simulink library "dynamic_capacity_server"  (R2019a)
settings: Solver=VariableStepAuto  StartTime=0.0  StopTime=10.0  RelTol=1e-3
undefined symbols (not defined in the file or in its folder): m, n
libraries: $bdroot x9
settings Model: Creator=arsineh  LastModifiedBy=arsineh

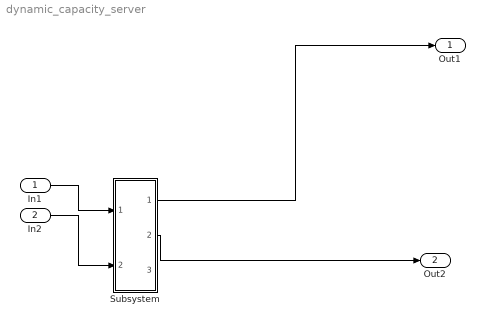
== system dynamic_capacity_server ==
  In1 : Inport
  In2 : Inport  Port=2
  Subsystem : Subsystem
  Out1 : Outport
  Out2 : Outport  Port=2
  wires:
  In1/1 -> Subsystem/1(In1)
  In2/1 -> Subsystem/2(In2)
  Subsystem/1(Out1) -> Out1/1
  Subsystem/2(Out2) -> Out2/1

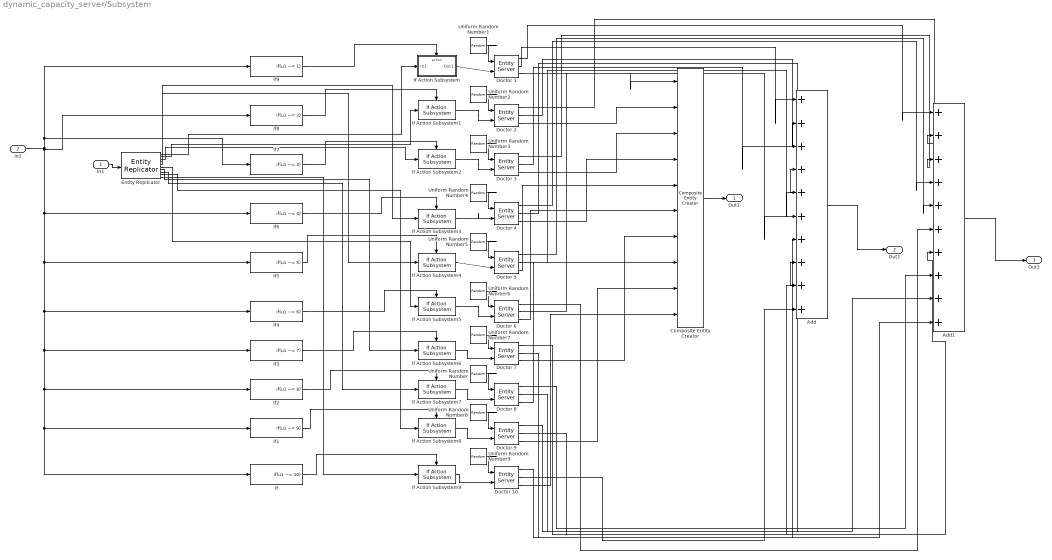
== system dynamic_capacity_server/Subsystem ==
  In1 : Inport
  In2 : Inport  Port=2
  Add : Sum  Inputs=++++++++++
  Add1 : Sum  Inputs=++++++++++
  Composite Entity Creator : CompositeEntityCreator  InputPortMessageModes=m,m,m,m,m,m,m,m,m,m  OutputPortMessageModes=m  NumberInputPorts=10  EntityTypeName=Combined
      settings: InputPortMap=u0,u1,u2,u3,u4,u5,u6,u7,u8,u9
  Doctor 1 : EntityServer  InputPortMessageModes=n,m  OutputPortMessageModes=n,n,m  Capacity=1  ServiceTimeSource=Signal port  ServiceTimeValue=30  ServiceTimeAction=dt = randi([30,60]);  NumberEntitiesDeparted=on  AverageWait=on
      settings: InputPortMap=u0,u2  OutputPortMap=o0,o4,o9
  Doctor 10 : EntityServer  InputPortMessageModes=n,m  OutputPortMessageModes=n,n,m  Capacity=10  ServiceTimeSource=Signal port  ServiceTimeValue=30  ServiceTimeAction=dt = randi([30,60]);  NumberEntitiesDeparted=on  AverageWait=on
      settings: InputPortMap=u0,u2  OutputPortMap=o0,o4,o9
  Doctor 2 : EntityServer  InputPortMessageModes=n,m  OutputPortMessageModes=n,n,m  Capacity=2  ServiceTimeSource=Signal port  ServiceTimeValue=30  ServiceTimeAction=dt = randi([30,60]);  NumberEntitiesDeparted=on  AverageWait=on
      settings: InputPortMap=u0,u2  OutputPortMap=o0,o4,o9
  Doctor 3 : EntityServer  InputPortMessageModes=n,m  OutputPortMessageModes=n,n,m  Capacity=3  ServiceTimeSource=Signal port  ServiceTimeValue=30  ServiceTimeAction=dt = randi([30,60]);  NumberEntitiesDeparted=on  AverageWait=on
      settings: InputPortMap=u0,u2  OutputPortMap=o0,o4,o9
  Doctor 4 : EntityServer  InputPortMessageModes=n,m  OutputPortMessageModes=n,n,m  Capacity=4  ServiceTimeSource=Signal port  ServiceTimeValue=30  ServiceTimeAction=dt = randi([30,60]);  NumberEntitiesDeparted=on  AverageWait=on
      settings: InputPortMap=u0,u2  OutputPortMap=o0,o4,o9
  Doctor 5 : EntityServer  InputPortMessageModes=n,m  OutputPortMessageModes=n,n,m  ServiceTimeSource=Signal port  ServiceTimeValue=30  ServiceTimeAction=dt = randi([30,60]);  NumberEntitiesDeparted=on  AverageWait=on
      settings: InputPortMap=u0,u2  OutputPortMap=o0,o4,o9
  Doctor 6 : EntityServer  InputPortMessageModes=n,m  OutputPortMessageModes=n,n,m  Capacity=6  ServiceTimeSource=Signal port  ServiceTimeValue=30  ServiceTimeAction=dt = randi([30,60]);  NumberEntitiesDeparted=on  AverageWait=on
      settings: InputPortMap=u0,u2  OutputPortMap=o0,o4,o9
  Doctor 7 : EntityServer  InputPortMessageModes=n,m  OutputPortMessageModes=n,n,m  Capacity=7  ServiceTimeSource=Signal port  ServiceTimeValue=30  ServiceTimeAction=dt = randi([30,60]);  NumberEntitiesDeparted=on  AverageWait=on
      settings: InputPortMap=u0,u2  OutputPortMap=o0,o4,o9
  Doctor 8 : EntityServer  InputPortMessageModes=n,m  OutputPortMessageModes=n,n,m  Capacity=8  ServiceTimeSource=Signal port  ServiceTimeValue=30  ServiceTimeAction=dt = randi([30,60]);  NumberEntitiesDeparted=on  AverageWait=on
      settings: InputPortMap=u0,u2  OutputPortMap=o0,o4,o9
  Doctor 9 : EntityServer  InputPortMessageModes=n,m  OutputPortMessageModes=n,n,m  Capacity=9  ServiceTimeSource=Signal port  ServiceTimeValue=30  ServiceTimeAction=dt = randi([30,60]);  NumberEntitiesDeparted=on  AverageWait=on
      settings: InputPortMap=u0,u2  OutputPortMap=o0,o4,o9
  Entity Replicator : EntityReplicator  InputPortMessageModes=m  OutputPortMessageModes=m,m,m,m,m,m,m,m,m,m  NumberReplicas=9
      settings: OutputPortMap=o0,o1,o2,o3,o4,o5,o6,o7,o8,o9
  If : If  IfExpression=u1 ~= 10  ShowElse=off
  If Action Subsystem : Subsystem  TreatAsAtomicUnit=on
  If Action Subsystem{1..9} (9 alike) : $bdroot/Subsystem/If Action Subsystem  SystemSampleTime=-1
  If1 : If  IfExpression=u1 ~= 9  ShowElse=off
  If2 : If  IfExpression=u1 ~= 8  ShowElse=off
  If3 : If  IfExpression=u1 ~= 7  ShowElse=off
  If4 : If  IfExpression=u1 ~= 6  ShowElse=off
  If5 : If  IfExpression=u1 ~= 5  ShowElse=off
  If6 : If  IfExpression=u1 ~= 4  ShowElse=off
  If7 : If  IfExpression=u1 ~= 3  ShowElse=off
  If8 : If  IfExpression=u1 ~= 2  ShowElse=off
  If9 : If  IfExpression=u1 ~= 1  ShowElse=off
  Uniform Random Number{,1..9} (10 alike) : UniformRandomNumber  Minimum=30  Maximum=60  Seed=234234234  SampleTime=0.1
  Out1 : Outport
  Out2 : Outport  Port=2
  Out3 : Outport  Port=3
  wires:
  Doctor 3/3 -> Composite Entity Creator/3
  Doctor 6/2 -> Add/6
  Doctor 6/3 -> Composite Entity Creator/6
  Doctor 9/2 -> Add/9
  Doctor 5/2 -> Add/5
  Doctor 9/3 -> Composite Entity Creator/9
  Doctor 7/3 -> Composite Entity Creator/7
  Entity Replicator/4 -> If Action Subsystem3/1
  Doctor 10/2 -> Add/10
  If Action Subsystem5/1 -> Doctor 6/2
  Uniform Random Number6/1 -> Doctor 6/1
  Doctor 2/2 -> Add/2
  Uniform Random Number/1 -> Doctor 8/1
  Entity Replicator/7 -> If Action Subsystem6/1
  If4/1 -> If Action Subsystem5/Action
  If5/1 -> If Action Subsystem4/Action
  Entity Replicator/5 -> If Action Subsystem4/1
  Doctor 2/3 -> Composite Entity Creator/2
  Doctor 8/3 -> Composite Entity Creator/8
  Doctor 7/2 -> Add/7
  If2/1 -> If Action Subsystem7/Action
  Entity Replicator/8 -> If Action Subsystem7/1
  Doctor 1/3 -> Composite Entity Creator/1
  If Action Subsystem1/1 -> Doctor 2/2
  Uniform Random Number5/1 -> Doctor 5/1
  Entity Replicator/6 -> If Action Subsystem5/1
  If Action Subsystem8/1 -> Doctor 9/2
  Doctor 10/3 -> Composite Entity Creator/10
  If1/1 -> If Action Subsystem8/Action
  Entity Replicator/2 -> If Action Subsystem1/1
  Entity Replicator/10 -> If Action Subsystem9/1
  Entity Replicator/3 -> If Action Subsystem2/1
  If Action Subsystem4/1 -> Doctor 5/2
  Uniform Random Number8/1 -> Doctor 9/1
  Doctor 4/3 -> Composite Entity Creator/4
  If9/1 -> If Action Subsystem/Action
  Doctor 1/2 -> Add/1
  Doctor 5/3 -> Composite Entity Creator/5
  If Action Subsystem2/1 -> Doctor 3/2
  Doctor 4/2 -> Add/4
  If Action Subsystem9/1 -> Doctor 10/2
  Uniform Random Number2/1 -> Doctor 2/1
  Entity Replicator/1 -> If Action Subsystem/1(In1)
  Entity Replicator/9 -> If Action Subsystem8/1
  If Action Subsystem3/1 -> Doctor 4/2
  Uniform Random Number3/1 -> Doctor 3/1
  Uniform Random Number7/1 -> Doctor 7/1
  If Action Subsystem7/1 -> Doctor 8/2
  If Action Subsystem/1(Out1) -> Doctor 1/2
  If/1 -> If Action Subsystem9/Action
  If3/1 -> If Action Subsystem6/Action
  Doctor 8/2 -> Add/8
  If Action Subsystem6/1 -> Doctor 7/2
  In1/1 -> Entity Replicator/1
  Doctor 3/2 -> Add/3
  Uniform Random Number4/1 -> Doctor 4/1
  Uniform Random Number9/1 -> Doctor 10/1
  Uniform Random Number1/1 -> Doctor 1/1
  Add/1 -> Out2/1
  Doctor 10/1 -> Add1/10
  Doctor 9/1 -> Add1/9
  Doctor 8/1 -> Add1/8
  Doctor 7/1 -> Add1/7
  Doctor 6/1 -> Add1/6
  Doctor 5/1 -> Add1/5
  Doctor 4/1 -> Add1/4
  Doctor 3/1 -> Add1/3
  Doctor 2/1 -> Add1/2
  Doctor 1/1 -> Add1/1
  Add1/1 -> Out3/1
  Composite Entity Creator/1 -> Out1/1
  If7/1 -> If Action Subsystem2/Action
  If6/1 -> If Action Subsystem3/Action
  If8/1 -> If Action Subsystem1/Action
  In2/1 -> If/1, If1/1, If2/1, If3/1, If4/1, If5/1, If6/1, If8/1, If7/1, If9/1

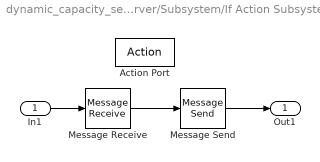
== system dynamic_capacity_server/Subsystem/If Action Subsystem ==
  In1 : Inport
  Action Port : ActionPort  ActionPortLabel=if(u1 ~= 1)
  Message Receive : MessageReceive  InputPortMessageModes=m
      settings: OutputPortMap=o1
  Message Send : MessageSend  OutputPortMessageModes=m
      settings: InputPortMap=u1
  Out1 : Outport
  wires:
  In1/1 -> Message Receive/1
  Message Receive/1 -> Message Send/1
  Message Send/1 -> Out1/1
